simulink model "Ship_PI"  (R2021a)
settings: Solver=VariableStepAuto  StartTime=0.0  StopTime=2000  RelTol=1e-3
values from neighbouring files (symbols this model uses):
  Bg = 1    [Run_Ship_PI.m]
  Bs = mean(B)    [Run_Ship_PI.m]
  Cg = 1    [Run_Ship_PI.m]
  Cs = abs(mean(C))    [Run_Ship_PI.m]
  Ig = 1    [Run_Ship_PI.m]
  Is = ((1/12)*2)+(0.5+0.6^2)    (= 1.02666666667)    [Run_Ship_PI.m]
  Kd = 600    [Run_Ship_PI.m]
  Kg = Wspin*Ispin    (= 1)    [Run_Ship_PI.m]
  Kp = 30    [Run_Ship_PI.m]
  w = 1    [Run_Ship_PI.m]
libraries: simulink x1
settings Model: Creator=samcl  LastModifiedBy=samcl

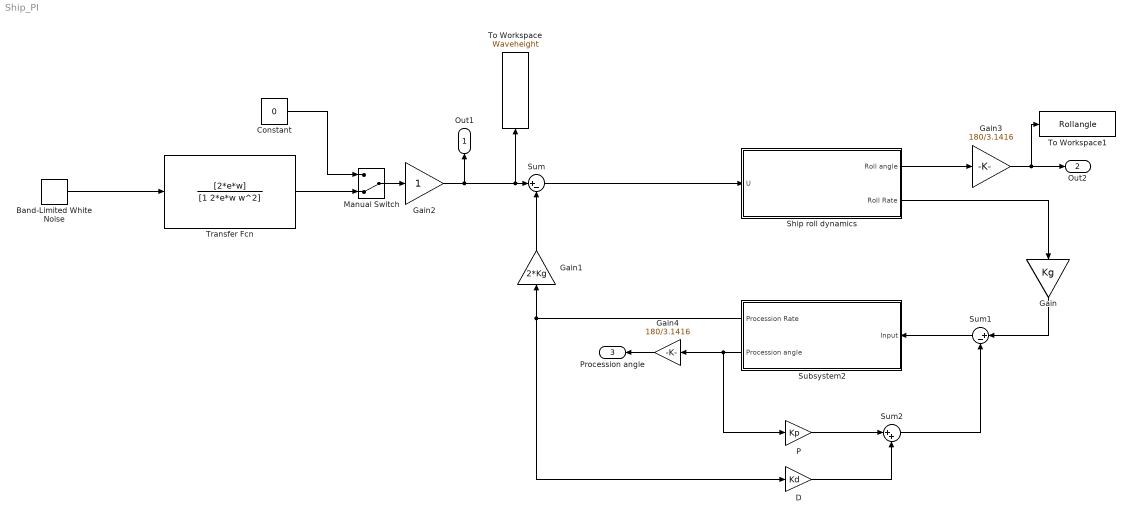
== system Ship_PI ==
  Band-Limited White Noise : simulink/Sources/Band-Limited White Noise  Cov=[0.1]  Ts=0.1  seed=[23341]
  Constant : Constant  Value=0
  D : Gain  Gain=Kd
  Gain : Gain  Gain=Kg
  Gain1 : Gain  Gain=2*Kg
  Gain2 : Gain
  Gain3 : Gain  Gain=180/3.1416
  Gain4 : Gain  Gain=180/3.1416
  Manual Switch : ManualSwitch  CurrentSetting=0
  P : Gain  Gain=Kp
  Ship roll dynamics : Subsystem  Description=plant
      settings: MinAlgLoopOccurrences=on
  Subsystem2 : Subsystem
  Sum : Sum  Inputs=|+-
  Sum1 : Sum  Inputs=|+-
  Sum2 : Sum  Inputs=|++
  To Workspace : ToWorkspace  VariableName=Waveheight  SampleTime=-1
  To Workspace1 : ToWorkspace  VariableName=Rollangle  SampleTime=-1
  Transfer Fcn : TransferFcn  Numerator=[2*e*w]  Denominator=[1 2*e*w w^2]
  Out1 : Outport  SignalName=Wave
  Out2 : Outport  Port=2  SignalName=Roll angle
  Procession angle : Outport  Port=3  SignalName=Gyro angle
  wires:
  Band-Limited White Noise/1 -> Transfer Fcn/1
  Sum2/1 -> Sum1/2
  Gain/1 -> Sum1/1
  Ship roll dynamics/1(Roll angle) -> Gain3/1
  Sum/1 -> Ship roll dynamics/1(U)
  Gain1/1 -> Sum/2
  P/1 -> Sum2/1
  D/1 -> Sum2/2
  Sum1/1 -> Subsystem2/1(Input)
  Subsystem2/1(Procession Rate) -> Gain1/1, D/1
  Subsystem2/2(Procession angle) -> Gain4/1, P/1
  Manual Switch/1 -> Gain2/1
  Transfer Fcn/1 -> Manual Switch/2
  Constant/1 -> Manual Switch/1
  Gain2/1 -> To Workspace/1, Sum/1, Out1/1
  Gain3/1 -> To Workspace1/1, Out2/1
  Ship roll dynamics/2(Roll Rate) -> Gain/1
  Gain4/1 -> Procession angle/1

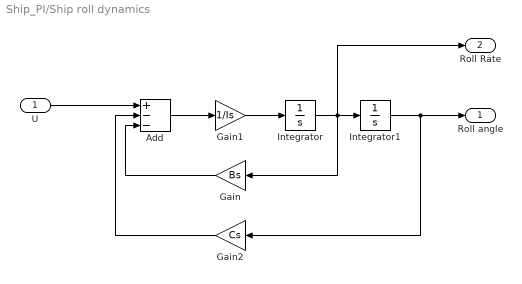
== system Ship_PI/Ship roll dynamics ==
  U : Inport
  Add : Sum  Inputs=+--
  Gain : Gain  Gain=Bs
  Gain1 : Gain  Gain=1/Is
  Gain2 : Gain  Gain=Cs
  Integrator : Integrator
  Integrator1 : Integrator
  Roll angle : Outport
  Roll Rate : Outport  Port=2
  wires:
  U/1 -> Add/1
  Add/1 -> Gain1/1
  Gain1/1 -> Integrator/1
  Integrator/1 -> Gain/1, Roll Rate/1, Integrator1/1
  Integrator1/1 -> Gain2/1, Roll angle/1
  Gain2/1 -> Add/2
  Gain/1 -> Add/3

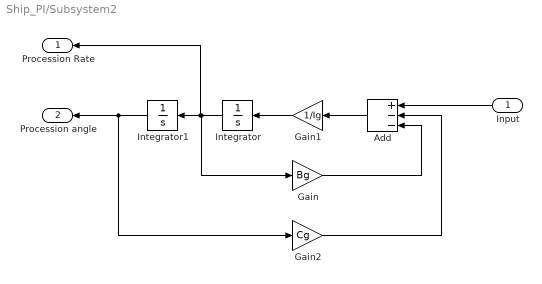
== system Ship_PI/Subsystem2 ==
  Input : Inport
  Add : Sum  Inputs=+--
  Gain : Gain  Gain=Bg
  Gain1 : Gain  Gain=1/Ig
  Gain2 : Gain  Gain=Cg
  Integrator : Integrator
  Integrator1 : Integrator
  Procession Rate : Outport
  Procession angle : Outport  Port=2
  wires:
  Input/1 -> Add/1
  Add/1 -> Gain1/1
  Integrator1/1 -> Procession angle/1, Gain2/1
  Gain/1 -> Add/3
  Gain2/1 -> Add/2
  Integrator/1 -> Procession Rate/1, Integrator1/1, Gain/1
  Gain1/1 -> Integrator/1
